simulink model "simpSimuRoboToGoRauschKalmanRegel"  (R2019b)
settings: Solver=FixedStepDiscrete  StartTime=0.0  StopTime=50.0  FixedStep=0.1  RelTol=1e-3  EnableMultiTasking=on
undefined symbols (not defined in the file): Discrete, Time
libraries: fahrradDiskr x1, ctrlSharedLib x1, simulink x1
settings Model: Creator=pic  LastModifiedBy=mackst
settings SolverCC: ZeroCrossAlgorithm=Adaptive
settings DataIOCC: SaveFormat=Array  TimeSaveName=t  OutputSaveName=y
settings OptimizationCC: ExpressionDepthLimit=2147483647  LifeSpan=inf
settings DebuggingCC: UnderspecifiedInitializationDetection=Classic  MergeDetectMultiDrivingBlocksExec=none  SolverPrmCheckMsg=warning  AllowSymbolicDim=off  StateNameClashWarn=warning  SFUnexpectedBacktrackingDiag=warning  SFNoUnconditionalDefaultTransitionDiag=warning  SFExecutionAtInitializationDiag=none  ArithmeticOperatorsInVariantConditions=warning
settings HardwareCC: ProdBitPerPointer=32  ProdBitPerSizeT=32  ProdBitPerPtrDiffT=32  ProdLargestAtomicFloat=None  ProdIntDivRoundTo=Undefined  ProdEndianess=Unspecified  ProdWordSize=32  ProdHWDeviceType=32-bit Generic
settings ModelReferenceCC: PropagateSignalLabelsOutOfModel=off
settings SFSimCC: SimUseLocalCustomCode=off  CustomCodeUndefinedFunction=UseInterfaceOnly
settings RTWCC: RTWUseLocalCustomCode=off
settings CodeAppCC: StateflowObjectComments=on
settings GRTTargetCC: TargetLangStandard=C89/C90 (ANSI)  GeneratePreprocessorConditionals=Disable all  CombineOutputUpdateFcns=off  GRTInterface=on
settings ConfigComp: CovMetricSettings=dw  CovHtmlReporting=on  CovSaveCumulativeToWorkspaceVar=on  CovSaveSingleToWorkspaceVar=on  CovExternalEMLEnable=off

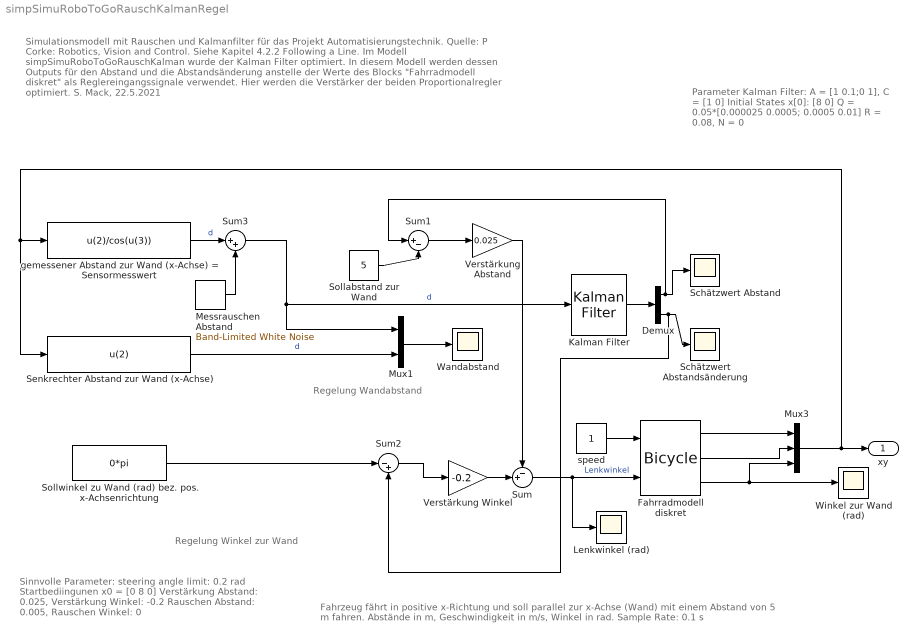
== system simpSimuRoboToGoRauschKalmanRegel ==
  note: Sinnvolle Parameter:
      | steering angle limit: 0.2 rad
      | Startbediingunen x0 = [0 8 0]
      | Verstärkung Abstand: 0.025, Verstärkung Winkel: -0.2
      | Rauschen Abstand: 0.005, Rauschen Winkel: 0
  note: Regelung Wandabstand
  note: Regelung Winkel zur Wand
  note: Simulationsmodell mit Rauschen und Kalmanfilter für das Projekt Automatisierungstechnik.
      | Quelle: P Corke: Robotics, Vision and Control. Siehe Kapitel 4.2.2 Following a Line.
      |
      | Im Modell simpSimuRoboToGoRauschKalman wurde der Kalman Filter optimiert. In diesem Modell werden dessen Outputs für den Abstand und
      | die Abstandsänderung anstelle der Werte des Blocks "Fahrradmodell diskret" als Reglereingangssignale verwendet.
      | Hier werden die Verstärker der beiden Proportionalregler optimiert.
      |
      | S. Mack, 22.5.2021
  note: Fahrzeug fährt in positive x-Richtung und soll parallel zur x-Achse (Wand) mit einem Abstand
      | von 5 m fahren. Abstände in m, Geschwindigkeit in m/s, Winkel in rad.
      | Sample Rate: 0.1 s
  note: Parameter Kalman Filter:
      | A = [1 0.1;0 1], C = [1 0]
      | Initial States x[0]: [8 0]
      | Q = 0.05*[0.000025 0.0005; 0.0005 0.01]
      | R = 0.08, N = 0
  Demux : Demux  Outputs=2
  Fahrradmodell diskret : fahrradDiskr/Vehicles/Bicycle  vlim=1  accel=Inf  alim=0.2  steer_rate=Inf  L=1  x0=[0, 8, 0]
  Kalman Filter : ctrlSharedLib/Kalman Filter  TimeDomain=Discrete-Time  UseCurrentEstimator=on  ModelSource=Individual A, B, C, D matrices  ModelSourceVariable=ss(0.95,1,1,0,1)  A=[1 0.1;0 1]  B=0  C=[1 0]  D=0  NumberOfStates=1  NumberOfInputs=1  NumberOfOutputs=1  InitialEstimateSource=Dialog  X0=[8 0]  P0=10  UseK=off  UseGH=off  NumberOfProcessNoiseInputs=1  G=1  TimeInvariantG=on  H=0  TimeInvariantH=on  Q=0.05*[0.000025 0.0005; 0.0005 0.01]  TimeInvariantQ=on  R=0.08  TimeInvariantR=on  N=0  TimeInvariantN=on  AddInputPort=off  AddEnablePort=off  OutputEstimatedY=off  OutputP=off  Ts=-1
      settings: SourceProductBaseCode=CT
  Lenkwinkel (rad) : Scope
  Messrauschen Abstand : simulink/Sources/Band-Limited White Noise  Cov=[0.005]  Ts=0.1  seed=[23341]
  Mux1 : Mux  Inputs=2
  Mux3 : Mux  Inputs=3
  Schätzwert Abstand : Scope
  Schätzwert Abstandsänderung : Scope
  Senkrechter Abstand zur Wand (x-Achse) : Fcn  Expr=u(2)
  Sollabstand zur Wand : Constant  Value=5
  Sollwinkel zu Wand (rad) bez. pos. x-Achsenrichtung : Constant  Value=0*pi
  Sum : Sum  Inputs=-+|
  Sum1 : Sum  Inputs=|+-
  Sum2 : Sum  Inputs=|-+
  Sum3 : Sum  Inputs=|++
  Verstärkung Abstand : Gain  Gain=0.025
  Verstärkung Winkel : Gain  Gain=-0.2
  Wandabstand : Scope
  Winkel zur Wand (rad) : Scope
  gemessener Abstand zur Wand (x-Achse) = Sensormesswert : Fcn  Expr=u(2)/cos(u(3))
  speed : Constant  VectorParams1D=off  SampleTime=-1
  xy : Outport  VectorParamsAs1DForOutWhenUnconnected=off
  wires:
  Mux3/1 -> xy/1, Senkrechter Abstand zur Wand (x-Achse)/1, gemessener Abstand zur Wand (x-Achse) = Sensormesswert/1
  Verstärkung Winkel/1 -> Sum/2
  speed/1 -> Fahrradmodell diskret/1
  Sum/1 -> Lenkwinkel (rad)/1, Fahrradmodell diskret/2  "Lenkwinkel"
  Fahrradmodell diskret/1 -> Mux3/1
  Fahrradmodell diskret/2 -> Mux3/2
  Fahrradmodell diskret/3 -> Winkel zur Wand (rad)/1, Mux3/3
  Verstärkung Abstand/1 -> Sum/1
  Sum1/1 -> Verstärkung Abstand/1
  Sollabstand zur Wand/1 -> Sum1/2
  Mux1/1 -> Wandabstand/1
  Sum3/1 -> Mux1/1, Kalman Filter/1  "d"
  Senkrechter Abstand zur Wand (x-Achse)/1 -> Mux1/2  "d"
  Sum2/1 -> Verstärkung Winkel/1
  Messrauschen Abstand/1 -> Sum3/2
  gemessener Abstand zur Wand (x-Achse) = Sensormesswert/1 -> Sum3/1  "d"
  Sollwinkel zu Wand (rad) bez. pos. x-Achsenrichtung/1 -> Sum2/1
  Kalman Filter/1 -> Demux/1
  Demux/1 -> Sum1/1, Schätzwert Abstand/1
  Demux/2 -> Sum2/2, Schätzwert Abstandsänderung/1
